simulink model "CP_ContrSys_Lin_a_n9558292"  (R2018a)
settings: Solver=VariableStepAuto  StartTime=0.0  StopTime=10.0  RelTol=1e-3
values from neighbouring files (symbols this model uses):
  Aa = [0,0,1,0;0,0,0,1;0,-m*g/Mc,0,0;0,g*(Mc+m)/(l*Mc),0,0]    [CP_ContrSys_Lin_a_MainFile_n9558292.m]    (also in CP_ContrSys_Lin_b_MainFile_n9558292.m = [0,0,1,0;0,0,0,1;0,-m*g/Mc,0,0;0,-g*(Mc+m)/(l*Mc),0,0])
  Ba = [0;0;1/Mc;-1/(l*Mc)]    [CP_ContrSys_Lin_a_MainFile_n9558292.m]    (also in CP_ContrSys_Lin_b_MainFile_n9558292.m = [0;0;1/Mc;1/(l*Mc)])
  Ca = [1,0,0,0;0,1,0,0]    [CP_ContrSys_Lin_a_MainFile_n9558292.m]    (also in CP_ContrSys_Lin_b_MainFile_n9558292.m)
  Ka = place(Aa,Ba,Pa)    [CP_ContrSys_Lin_a_MainFile_n9558292.m]    (also in CP_ContrSys_Lin_b_MainFile_n9558292.m)
  La = place(Aa',Ca',PLa)'    [CP_ContrSys_Lin_a_MainFile_n9558292.m]    (also in CP_ContrSys_Lin_b_MainFile_n9558292.m)
  x10 = 0.2    [CP_ContrSys_Lin_a_MainFile_n9558292.m]    (also in CP_ContrSys_Lin_b_MainFile_n9558292.m)
  x20 = deg2rad(20)    [CP_ContrSys_Lin_a_MainFile_n9558292.m]    (also in CP_ContrSys_Lin_b_MainFile_n9558292.m = deg2rad(200))
  x30 = 0    [CP_ContrSys_Lin_a_MainFile_n9558292.m]    (also in CP_ContrSys_Lin_b_MainFile_n9558292.m)
  x40 = 0    [CP_ContrSys_Lin_a_MainFile_n9558292.m]    (also in CP_ContrSys_Lin_b_MainFile_n9558292.m)
settings Model: Creator=haidarobeid  LastModifiedBy=haidarobeid

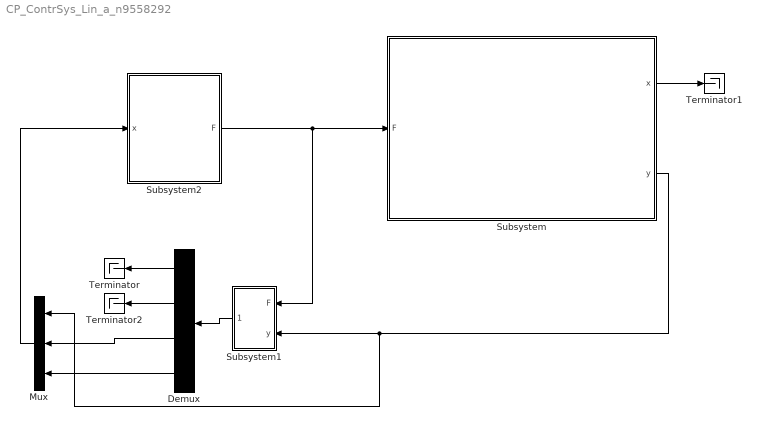
== system CP_ContrSys_Lin_a_n9558292 ==
  Demux : Demux
  Mux : Mux  Inputs=3
  Subsystem : Subsystem
  Subsystem1 : Subsystem
  Subsystem2 : Subsystem
  Terminator : Terminator
  Terminator1 : Terminator
  Terminator2 : Terminator
  wires:
  Subsystem/2(y) -> Mux/1, Subsystem1/2(y)
  Subsystem2/1(F) -> Subsystem1/1(F), Subsystem/1(F)
  Subsystem/1(x) -> Terminator1/1
  Demux/1 -> Terminator/1
  Subsystem1/1(xhat) -> Demux/1
  Demux/2 -> Terminator2/1
  Demux/3 -> Mux/2
  Demux/4 -> Mux/3
  Mux/1 -> Subsystem2/1(x)

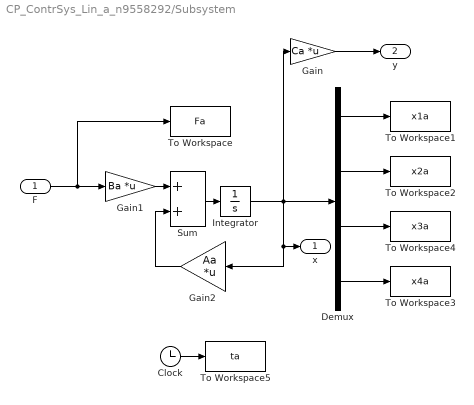
== system CP_ContrSys_Lin_a_n9558292/Subsystem ==
  F : Inport
  Clock : Clock
  Demux : Demux
  Gain : Gain  Gain=Ca  Multiplication=Matrix(K*u)
  Gain1 : Gain  Gain=Ba  Multiplication=Matrix(K*u)
  Gain2 : Gain  Gain=Aa  Multiplication=Matrix(K*u)
  Integrator : Integrator  InitialCondition=[x10,x20,x30,x40]'
  Sum : Sum
  To Workspace : ToWorkspace  VariableName=Fa  SampleTime=-1
  To Workspace1 : ToWorkspace  VariableName=x1a  SampleTime=-1
  To Workspace2 : ToWorkspace  VariableName=x2a  SampleTime=-1
  To Workspace3 : ToWorkspace  VariableName=x4a  SampleTime=-1
  To Workspace4 : ToWorkspace  VariableName=x3a  SampleTime=-1
  To Workspace5 : ToWorkspace  VariableName=ta  SampleTime=-1
  x : Outport
  y : Outport  Port=2
  wires:
  Demux/3 -> To Workspace4/1
  Demux/2 -> To Workspace2/1
  Demux/4 -> To Workspace3/1
  F/1 -> Gain1/1, To Workspace/1
  Demux/1 -> To Workspace1/1
  Clock/1 -> To Workspace5/1
  Gain/1 -> y/1
  Integrator/1 -> Gain2/1, x/1, Gain/1, Demux/1
  Gain1/1 -> Sum/1
  Sum/1 -> Integrator/1
  Gain2/1 -> Sum/2

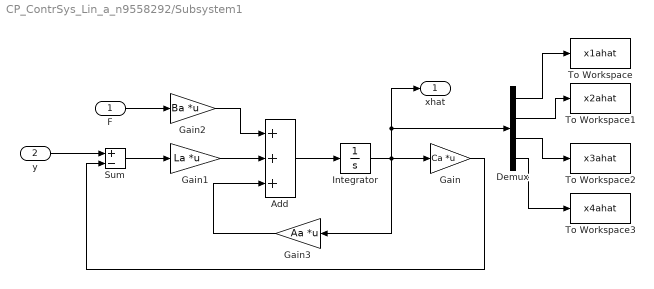
== system CP_ContrSys_Lin_a_n9558292/Subsystem1 ==
  F : Inport
  y : Inport  Port=2
  Add : Sum  Inputs=+++
  Demux : Demux
  Gain : Gain  Gain=Ca  Multiplication=Matrix(K*u)
  Gain1 : Gain  Gain=La  Multiplication=Matrix(K*u)
  Gain2 : Gain  Gain=Ba  Multiplication=Matrix(K*u)
  Gain3 : Gain  Gain=Aa  Multiplication=Matrix(K*u)
  Integrator : Integrator
  Sum : Sum  Inputs=+-
  To Workspace : ToWorkspace  VariableName=x1ahat  SampleTime=-1
  To Workspace1 : ToWorkspace  VariableName=x2ahat  SampleTime=-1
  To Workspace2 : ToWorkspace  VariableName=x3ahat  SampleTime=-1
  To Workspace3 : ToWorkspace  VariableName=x4ahat  SampleTime=-1
  xhat : Outport
  wires:
  Demux/1 -> To Workspace/1
  Demux/3 -> To Workspace2/1
  Gain2/1 -> Add/1
  y/1 -> Sum/1
  Integrator/1 -> xhat/1, Demux/1, Gain3/1, Gain/1
  Gain1/1 -> Add/2
  Add/1 -> Integrator/1
  Gain3/1 -> Add/3
  Sum/1 -> Gain1/1
  Demux/2 -> To Workspace1/1
  Gain/1 -> Sum/2
  F/1 -> Gain2/1
  Demux/4 -> To Workspace3/1

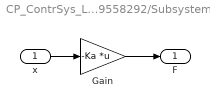
== system CP_ContrSys_Lin_a_n9558292/Subsystem2 ==
  x : Inport
  Gain : Gain  Gain=-Ka  Multiplication=Matrix(K*u)
  F : Outport
  wires:
  Gain/1 -> F/1
  x/1 -> Gain/1
